simulink model "mmcs_s2f"  (R2021b)
settings: Solver=FixedStepDiscrete  StartTime=0.0  StopTime=5  FixedStep=T_HF_TASK  RelTol=1e-3  EnableMultiTasking=on
PostLoadFcn:
  | run('init.m')
values from neighbouring files (symbols this model uses):
  ALIGN_DURATION = 700.0    [mmcs_s2f_dd.sldd]
  ALIGN_FINAL_CURRENT = 3277.0    [mmcs_s2f_dd.sldd]
  ALIGN_FINAL_SPEED = 0.0    [mmcs_s2f_dd.sldd]
  ALIGN_INIT_CURRENT = 1638.0    [mmcs_s2f_dd.sldd]
  ALIGN_THETA = 2731.0    [mmcs_s2f_dd.sldd]
  AMPTOS16 = 3277.0    [mmcs_s2f_dd.sldd]
  DIVSQRT_3 = 18918.0    [mmcs_s2f_dd.sldd]
  ENC_PT_CTRL = 4.0    [mmcs_s2f_dd.sldd]
  ENC_PULSE_NUM = 4000    [mmcs_s2f_dd.sldd]
  ENC_ST_CTRL = 2.0    [mmcs_s2f_dd.sldd]
  IF_ACC_DURATION = 1500.0    [mmcs_s2f_dd.sldd]
  IF_FINAL_CURRENT = 3277.0    [mmcs_s2f_dd.sldd]
  IF_FINAL_CURRENT_LOL = -3277.0    [mmcs_s2f_dd.sldd]
  IF_FINAL_CURRENT_UPL = 3277.0    [mmcs_s2f_dd.sldd]
  IF_FINAL_SPEED = 600.0    [mmcs_s2f_dd.sldd]
  IF_FINAL_SPEED_LOL = -600.0    [mmcs_s2f_dd.sldd]
  IF_FINAL_SPEED_UPL = 600.0    [mmcs_s2f_dd.sldd]
  IF_INIT_CURRENT = 1638.0    [mmcs_s2f_dd.sldd]
  INT16_MAX = 32767.0    [mmcs_s2f_dd.sldd]
  INT16_MIN = -32768.0    [mmcs_s2f_dd.sldd]
  MOTOR_F = 7.0E-6    [mmcs_s2f_dd.sldd]
  MOTOR_J = 2.8E-6    [mmcs_s2f_dd.sldd]
  MOTOR_PN = 4    [mmcs_s2f_dd.sldd]
  MOTOR_PNF = 4.0    [mmcs_s2f_dd.sldd]
  MOTOR_TL = 0.001    [mmcs_s2f_dd.sldd]
  PI_KI_PLL : value not decoded    [mmcs_s2f_dd.sldd]
  PI_KI_POS : value not decoded    [mmcs_s2f_dd.sldd]
  PI_KI_SPD : value not decoded    [mmcs_s2f_dd.sldd]
  PI_KI_TQ : value not decoded    [mmcs_s2f_dd.sldd]
  PI_KP_PLL : value not decoded    [mmcs_s2f_dd.sldd]
  PI_KP_POS : value not decoded    [mmcs_s2f_dd.sldd]
  PI_KP_SPD : value not decoded    [mmcs_s2f_dd.sldd]
  PI_KP_TQ : value not decoded    [mmcs_s2f_dd.sldd]
  PWM_FREQUENCY = 10000.0    [mmcs_s2f_dd.sldd]
  PWM_PERIOD_CYCLES = 7200.0    [mmcs_s2f_dd.sldd]
  RAD2RPM_F_DEN = 1000.0    [mmcs_s2f_dd.sldd]
  RAD2RPM_F_NUM = 9549.0    [mmcs_s2f_dd.sldd]
  RADTOS16_F = 10430.378350470453    [mmcs_s2f_dd.sldd]
  RADTOS16_I = 10430.0    [mmcs_s2f_dd.sldd]
  REF_CURRENT_LOL = -11470.0    [mmcs_s2f_dd.sldd]
  REF_CURRENT_UPL = 11470.0    [mmcs_s2f_dd.sldd]
  STM_ALIGN = 4.0    [mmcs_s2f_dd.sldd]
  STM_IFRUN = 5.0    [mmcs_s2f_dd.sldd]
  STM_INIT = 1.0    [mmcs_s2f_dd.sldd]
  STM_PTRUN = 7.0    [mmcs_s2f_dd.sldd]
  STM_START = 12.0    [mmcs_s2f_dd.sldd]
  STM_STRUN = 6.0    [mmcs_s2f_dd.sldd]
  STM_SWITCH = 11.0    [mmcs_s2f_dd.sldd]
  STO_C1 = 588    [mmcs_s2f_dd.sldd]
  STO_C2 = -5703    [mmcs_s2f_dd.sldd]
  STO_C3 = 1554    [mmcs_s2f_dd.sldd]
  STO_C4 = 7484    [mmcs_s2f_dd.sldd]
  STO_C5 = 1831    [mmcs_s2f_dd.sldd]
  STO_EST_MAX = 134213632.0    [mmcs_s2f_dd.sldd]
  STO_EST_MIN = -134213632.0    [mmcs_s2f_dd.sldd]
  STO_F1 = 4096.0    [mmcs_s2f_dd.sldd]
  STO_F2 = 4096.0    [mmcs_s2f_dd.sldd]
  STO_ST_CTRL = 3.0    [mmcs_s2f_dd.sldd]
  STOMS = 1000.0    [mmcs_s2f_dd.sldd]
  T_HF_TASK = 0.0001    [mmcs_s2f_dd.sldd]
  T_MF_TASK = 0.002    [mmcs_s2f_dd.sldd]
  TORQ_CTRL = 0.0    [mmcs_s2f_dd.sldd]
  U32MAXdivPulseNumber = 1073741    [mmcs_s2f_dd.sldd]
  VBUS = 24.0    [mmcs_s2f_dd.sldd]
undefined symbols (not defined in the file or in its folder): DiscIntNeverNeededParam
libraries: simulink x22, slpidlib x5, mcbplantlib x1, autolibpmsmexterior x1
(part 4 of 5)

== system mmcs_s2f/MFTask/SpdCtrl/SpdControler ==
  reset : Inport  OutDataTypeStr=boolean
  spd_ref : Inport  Port=2
  spd_fed : Inport  Port=3
  Constant6 : Constant  Value=0  OutDataTypeStr=int16
  Data Type Conversion : DataTypeConversion  OutDataTypeStr=int16  RndMeth=Zero
  Scope : Scope  NumInputPorts=2
  SpdControler : slpidlib/PID Controller  Controller=PI  Form=Parallel  TimeDomain=Discrete-time  UseExternalTs=off  SampleTime=-1  IntegratorMethod=Forward Euler  FilterMethod=Forward Euler  ControllerParametersSource=internal  P=PI_KP_SPD  I=PI_KI_SPD  D=0  UseFilter=on  N=100  TunerSelectOption=Transfer Function Based (PID Tuner App)  InitialConditionSource=internal  InitialConditionForIntegrator=0  InitialConditionForFilter=0  DifferentiatorICPrevScaledInput=0  ExternalReset=level  TrackingMode=off  Kt=1  LimitOutput=on  SatLimitsSource=internal  UpperSaturationLimit=REF_CURRENT_UPL  LowerSaturationLimit=REF_CURRENT_LOL  LinearizeAsGain=off  AntiWindupMode=clamping  Kb=1  RndMeth=Zero  SaturateOnIntegerOverflow=on  PGainOutDataTypeStr=fixdt(1,32,11)  PProdOutDataTypeStr=fixdt(1,32,11)  POutMin=[]  POutMax=[]  IGainOutDataTypeStr=fixdt(1,32,11)  IProdOutDataTypeStr=fixdt(1,32,11)  IOutMin=[]  IOutMax=[]  DOutMin=[]  DOutMax=[]  NOutMin=[]  NOutMax=[]  SumOutDataTypeStr=int32  SumOutMin=[]  SumOutMax=[]  SaturationOutDataTypeStr=int32  SaturationOutMin=[]  SaturationOutMax=[]  PParamDataTypeStr=fixdt(1,32,16)  PParamMin=[]  PParamMax=[]  IParamDataTypeStr=fixdt(1,32,16)  IParamMin=[]  IParamMax=[]  DParamMin=[]  DParamMax=[]  NParamMin=[]  NParamMax=[]  KbParamMin=[]  KbParamMax=[]  KtParamMin=[]  KtParamMax=[]  KbOutMin=[]  KbOutMax=[]  KtOutMin=[]  KtOutMax=[]  IntegratorOutDataTypeStr=fixdt(1,32,11)  IntegratorOutMin=[]  IntegratorOutMax=[]  FilterOutMin=[]  FilterOutMax=[]  SumI1OutMin=[]  SumI1OutMax=[]  SumI2OutMin=[]  SumI2OutMax=[]  SumI3OutMin=[]  SumI3OutMax=[]  SumI4OutMin=[]  SumI4OutMax=[]  SumDOutMin=[]  SumDOutMax=[]  SumAccumDataTypeStr=fixdt(1,32,11)  DifferentiatorOutMin=[]  DifferentiatorOutMax=[]  FilterDiffOutCoefMin=[]  FilterDiffOutCoefMax=[]  ReciprocalOutMin=[]  ReciprocalOutMax=[]  SumDenOutMin=[]  SumDenOutMax=[]  SumNumOutMin=[]  SumNumOutMax=[]  DivideOutMin=[]  DivideOutMax=[]  UdiffTsProdOutMin=[]  UdiffTsProdOutMax=[]  NTsProdOutMin=[]  NTsProdOutMax=[]  UintegralTsProdOutMin=[]  UintegralTsProdOutMax=[]  UngainTsProdOutMin=[]  UngainTsProdOutMax=[]  IntegratorContinuousStateAttributes=''  IntegratorStateMustResolveToSignalObject=off  IntegratorRTWStateStorageClass=Auto  FilterContinuousStateAttributes=''  FilterStateMustResolveToSignalObject=off  FilterRTWStateStorageClass=Auto  ParallelPVariant=InternalParameters  IdealPVariant=Disabled  IVariant=InternalParameters  DVariant=Disabled  IntegratorVariant=Discrete  SatVariant=Enabled  AWVariant=DiscClampingParallel  PCopyVariant=Disabled  TRVariant=Disabled  FdbkBlocksVariant=Forward  IdealPFdbkVariant=Disabled  SatFdbkVariant=Disabled  DerivativeFilterVariant=Disabled  NVariant=Disabled  NCopyVariant=Disabled_SignalSpec  FilterICVariant=Disabled  IntegratorICVariant=InternalICs  ExternalResetVariant=ExternalReset  TRSumVariant=Passthrough  SumFdbkVariant=Disabled  SumVariant=Sum_PI  TsampFilterVariant=InternalTs  TsampNgainVariant=Passthrough  TsampIntegralVariant=Passthrough  ExternalSaturationOutDataTypeStr=Inherit: Same as second input
  Sum : Sum  Inputs=|+-  RndMeth=Zero
  id_ref : Outport  OutDataTypeStr=int16
  iq_ref : Outport  Port=2  OutDataTypeStr=int16
  spd_ramp : Outport  Port=3  OutDataTypeStr=int16
  wires:
  Constant6/1 -> id_ref/1
  Sum/1 -> SpdControler/1
  spd_ref/1 -> Scope/1, spd_ramp/1, Sum/1
  spd_fed/1 -> Sum/2, Scope/2
  SpdControler/1 -> Data Type Conversion/1
  Data Type Conversion/1 -> iq_ref/1
  reset/1 -> SpdControler/2

== system mmcs_s2f/MFTask/SysCtrlModeUpdDet/If Action Subsystem ==
  pos_fed : Inport  OutDataTypeStr=int32
  Action Port : ActionPort  ActionPortLabel=if(u1)
  Constant : Constant  Value=0  OutDataTypeStr=uint8
  Constant1 : Constant  Value=0  OutDataTypeStr=single
  Constant2 : Constant  Value=RADTOS16_F  OutDataTypeStr=single
  Data Store Write1 : DataStoreWrite  DataStoreName=pos_ctrl  DataStoreElements=pos_ctrl.final_angle#pos_ctrl.theta#pos_ctrl.tc_sts#pos_ctrl.elapse_time  IndexOptions=Index vector (dialog)  Indices=1  OutputSizes=1
  Divide : Product  Inputs=*/  OutDataTypeStr=single  RndMeth=Zero
  wires:
  pos_fed/1 -> Divide/1
  Constant/1 -> Data Store Write1/3
  Constant1/1 -> Data Store Write1/4
  Constant2/1 -> Divide/2
  Divide/1 -> Data Store Write1/2, Data Store Write1/1

== system mmcs_s2f/MFTask/TorqCtrl/AlignRamp ==
  reset : Inport  OutDataTypeStr=uint8
  Constant1 : Constant  Value=ALIGN_INIT_CURRENT  OutDataTypeStr=int16
  Constant5 : Constant  Value=ALIGN_FINAL_CURRENT  OutDataTypeStr=int16
  Constant6 : Constant  Value=0  OutDataTypeStr=int16
  Constant7 : Constant  Value=ALIGN_DURATION  OutDataTypeStr=uint16
  Constant9 : Constant  Value=ALIGN_FINAL_SPEED  OutDataTypeStr=int16
  IfControler : Subsystem
      settings: RTWFcnNameOpts=Use subsystem name  RTWFileNameOpts=Use subsystem name
  id_ref : Outport  OutDataTypeStr=int16
  iq_ref : Outport  Port=2  OutDataTypeStr=int16
  spd_ramp : Outport  Port=3  OutDataTypeStr=int16
  wires:
  IfControler/1(i_ref) -> id_ref/1
  Constant7/1 -> IfControler/4(duration_ms)
  Constant9/1 -> IfControler/3(final_spd)
  Constant6/1 -> iq_ref/1
  Constant5/1 -> IfControler/2(final_i)
  reset/1 -> IfControler/5(reset)
  Constant1/1 -> IfControler/1(init_i)
  IfControler/2(spd_ref) -> spd_ramp/1

== system mmcs_s2f/MFTask/TorqCtrl/AligntAction ==
  id_ref_i : Inport  OutDataTypeStr=int16
  iq_ref_i : Inport  Port=2  OutDataTypeStr=int16
  spd_ramp_i : Inport  Port=3  OutDataTypeStr=int16
  Action Port : ActionPort  ActionPortLabel=case [ 4 ]:
  id_ref : Outport  OutDataTypeStr=int16
  iq_ref : Outport  Port=2  OutDataTypeStr=int16
  spd_ramp : Outport  Port=3  OutDataTypeStr=int16
  wires:
  id_ref_i/1 -> id_ref/1
  spd_ramp_i/1 -> spd_ramp/1
  iq_ref_i/1 -> iq_ref/1

== system mmcs_s2f/MFTask/TorqCtrl/DefAction ==
  Action Port : ActionPort  ActionPortLabel=default:
  Constant : Constant  Value=0  OutDataTypeStr=int16
  Constant1 : Constant  Value=0  OutDataTypeStr=int16
  Constant2 : Constant  Value=0  OutDataTypeStr=int16
  id_ref : Outport  OutDataTypeStr=int16
  iq_ref : Outport  Port=2  OutDataTypeStr=int16
  spd_ramp : Outport  Port=3  OutDataTypeStr=int16
  wires:
  Constant2/1 -> spd_ramp/1
  Constant1/1 -> iq_ref/1
  Constant/1 -> id_ref/1

== system mmcs_s2f/MFTask/TorqCtrl/IFRamp ==
  reset : Inport  OutDataTypeStr=uint8
  spd_ref : Inport  Port=2  OutDataTypeStr=int16
  Constant1 : Constant  Value=IF_INIT_CURRENT  OutDataTypeStr=int16
  Constant5 : Constant  Value=IF_FINAL_CURRENT  OutDataTypeStr=int16
  Constant6 : Constant  Value=0  OutDataTypeStr=int16
  Constant7 : Constant  Value=IF_ACC_DURATION  OutDataTypeStr=uint16
  Constant9 : Constant  Value=IF_FINAL_SPEED  OutDataTypeStr=int16
  Demux : Demux  Outputs=3
      settings: DisplayOption=none
  Gain : Gain  Gain=-1  ParamDataTypeStr=int16  OutDataTypeStr=int16  RndMeth=Zero
  IfControler : Subsystem
      settings: RTWFcnNameOpts=Use subsystem name  RTWFileNameOpts=Use subsystem name
  Mux : Mux  Inputs=3
  Switch : Switch  RndMeth=Zero
  id_ref : Outport  OutDataTypeStr=int16
  iq_ref : Outport  Port=2  OutDataTypeStr=int16
  spd_ramp : Outport  Port=3  OutDataTypeStr=int16
  wires:
  spd_ref/1 -> Switch/2
  IfControler/2(spd_ref) -> spd_ramp/1
  Constant6/1 -> id_ref/1
  IfControler/1(i_ref) -> iq_ref/1
  Constant7/1 -> IfControler/4(duration_ms)
  reset/1 -> IfControler/5(reset)
  Gain/1 -> Switch/3
  Constant1/1 -> Mux/1
  Constant5/1 -> Mux/2
  Constant9/1 -> Mux/3
  Mux/1 -> Gain/1, Switch/1
  Switch/1 -> Demux/1
  Demux/2 -> IfControler/2(final_i)
  Demux/1 -> IfControler/1(init_i)
  Demux/3 -> IfControler/3(final_spd)

== system mmcs_s2f/MFTask/TorqCtrl/IFStart ==
  id_ref_i : Inport  OutDataTypeStr=int16
  iq_ref_i : Inport  Port=2  OutDataTypeStr=int16
  spd_ramp_i : Inport  Port=3  OutDataTypeStr=int16
  Action Port : ActionPort  ActionPortLabel=case [ 5 ]:
  id_ref : Outport  OutDataTypeStr=int16
  iq_ref : Outport  Port=2  OutDataTypeStr=int16
  spd_ramp : Outport  Port=3  OutDataTypeStr=int16
  wires:
  iq_ref_i/1 -> iq_ref/1
  spd_ramp_i/1 -> spd_ramp/1
  id_ref_i/1 -> id_ref/1

== system mmcs_s2f/HFTask/AngleCalc/VssCalcAngle/EncCalcAngle ==
  cnt : Inport  OutDataTypeStr=int32
  Constant : Constant  Value=65536  OutDataTypeStr=int32
  Constant6 : Constant  Value=U32MAXdivPulseNumber  OutDataTypeStr=uint32
  Data Type Conversion1 : DataTypeConversion  OutDataTypeStr=int16  RndMeth=Zero
  Data Type Conversion2 : DataTypeConversion  OutDataTypeStr=int16  RndMeth=Zero
  Divide : Product  Inputs=*/  OutDataTypeStr=int32  RndMeth=Zero
  Gain5 : Gain  Gain=MOTOR_PN  OutDataTypeStr=int32  RndMeth=Zero
  Product2 : Product  OutDataTypeStr=int64  RndMeth=Zero
  Scope : Scope  NumInputPorts=2
  theta_e : Outport  OutDataTypeStr=int16
  wires:
  Constant6/1 -> Product2/2
  Product2/1 -> Divide/1
  Data Type Conversion2/1 -> Scope/2, theta_e/1  "theta_e"
  cnt/1 -> Product2/1
  Constant/1 -> Divide/2
  Divide/1 -> Data Type Conversion1/1
  Gain5/1 -> Data Type Conversion2/1
  Data Type Conversion1/1 -> Scope/1, Gain5/1  "theta_m"

== system mmcs_s2f/HFTask/AngleCalc/VssCalcAngle/VssEncoder ==
  spd_ref : Inport  OutDataTypeStr=int16
  theta_0 : Inport  Port=2  OutDataTypeStr=int16
  reset : Inport  Port=3  OutDataTypeStr=uint8
  Add : Sum  RndMeth=Zero
  Constant1 : Constant  Value=60  OutDataTypeStr=uint8
  Constant7 : Constant  Value=ENC_PULSE_NUM  OutDataTypeStr=int32
  Discrete-Time Integrator1 : DiscreteIntegrator  ExternalReset=level  SampleTime=-1  OutDataTypeStr=int32  RndMeth=Zero  ICPrevOutput=DiscIntNeverNeededParam  ICPrevScaledInput=DiscIntNeverNeededParam
  Divide : Product  Inputs=*/  OutDataTypeStr=int32  RndMeth=Zero
  Math Function : Math  Operator=rem  SaturateOnIntegerOverflow=on
  Product1 : Product  OutDataTypeStr=int32  RndMeth=Zero
  enc_cnt : Outport
  wires:
  spd_ref/1 -> Product1/1
  Constant7/1 -> Product1/2, Math Function/2
  Product1/1 -> Discrete-Time Integrator1/1
  Math Function/1 -> enc_cnt/1
  Discrete-Time Integrator1/1 -> Divide/1
  Divide/1 -> Add/1
  Add/1 -> Math Function/1
  theta_0/1 -> Add/2
  Constant1/1 -> Divide/2
  reset/1 -> Discrete-Time Integrator1/2

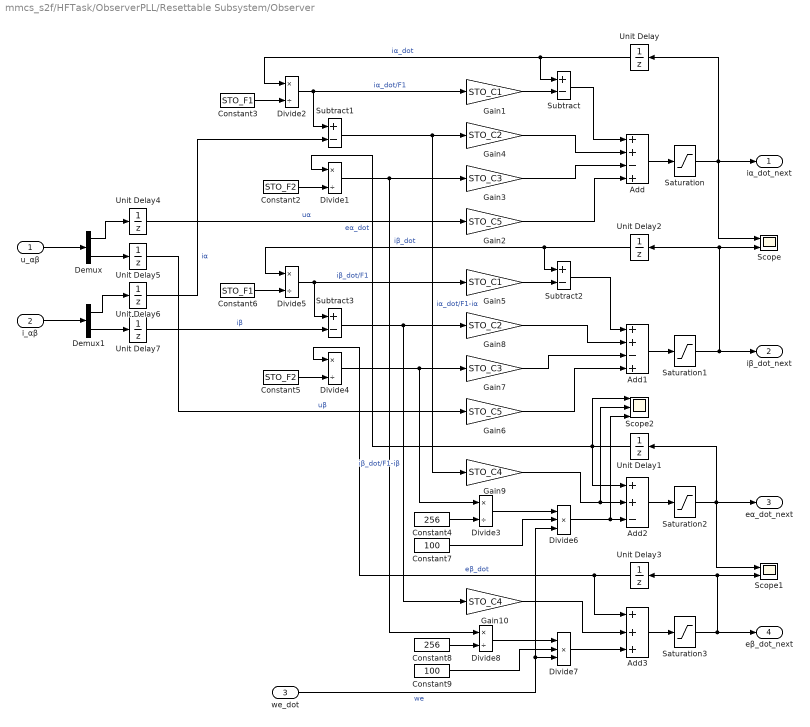
== system mmcs_s2f/HFTask/ObserverPLL/Resettable Subsystem/Observer ==
  u_αβ : Inport  OutDataTypeStr=int16
  i_αβ : Inport  Port=2  OutDataTypeStr=int16
  we_dot : Inport  Port=3  OutDataTypeStr=int16
  Add : Sum  Inputs=++-+  OutDataTypeStr=int32  RndMeth=Zero
  Add1 : Sum  Inputs=++-+  OutDataTypeStr=int32  RndMeth=Zero
  Add2 : Sum  Inputs=++-  OutDataTypeStr=int32  RndMeth=Zero
  Add3 : Sum  Inputs=+++  OutDataTypeStr=int32  RndMeth=Zero
  Constant2 : Constant  Value=STO_F2  OutDataTypeStr=int16
  Constant3 : Constant  Value=STO_F1  OutDataTypeStr=int16
  Constant4 : Constant  Value=256  OutDataTypeStr=int16
  Constant5 : Constant  Value=STO_F2  OutDataTypeStr=int16
  Constant6 : Constant  Value=STO_F1  OutDataTypeStr=int16
  Constant7 : Constant  Value=100  OutDataTypeStr=int16
  Constant8 : Constant  Value=256  OutDataTypeStr=int16
  Constant9 : Constant  Value=100  OutDataTypeStr=int16
  Demux : Demux  Outputs=2
      settings: DisplayOption=none
  Demux1 : Demux  Outputs=2
      settings: DisplayOption=none
  Divide{1..5,8} (6 alike) : Product  Inputs=*/  OutDataTypeStr=int32  RndMeth=Zero
  Divide6 : Product  Inputs=***  OutDataTypeStr=int32  RndMeth=Zero
  Divide7 : Product  Inputs=***  OutDataTypeStr=int32  RndMeth=Zero
  Gain1 : Gain  Gain=STO_C1  ParamDataTypeStr=int32  OutDataTypeStr=int32  RndMeth=Zero
  Gain10 : Gain  Gain=STO_C4  ParamDataTypeStr=int32  OutDataTypeStr=int32  RndMeth=Zero
  Gain2 : Gain  Gain=STO_C5  ParamDataTypeStr=int32  OutDataTypeStr=int32  RndMeth=Zero
  Gain3 : Gain  Gain=STO_C3  ParamDataTypeStr=int32  OutDataTypeStr=int32  RndMeth=Zero
  Gain4 : Gain  Gain=STO_C2  ParamDataTypeStr=int32  OutDataTypeStr=int32  RndMeth=Zero
  Gain5 : Gain  Gain=STO_C1  ParamDataTypeStr=int32  OutDataTypeStr=int32  RndMeth=Zero
  Gain6 : Gain  Gain=STO_C5  ParamDataTypeStr=int32  OutDataTypeStr=int32  RndMeth=Zero
  Gain7 : Gain  Gain=STO_C3  ParamDataTypeStr=int32  OutDataTypeStr=int32  RndMeth=Zero
  Gain8 : Gain  Gain=STO_C2  ParamDataTypeStr=int32  OutDataTypeStr=int32  RndMeth=Zero
  Gain9 : Gain  Gain=STO_C4  ParamDataTypeStr=int32  OutDataTypeStr=int32  RndMeth=Zero
  Saturation{,1..3} (4 alike) : Saturate  UpperLimit=STO_EST_MAX  LowerLimit=STO_EST_MIN  RndMeth=Zero
  Scope : Scope  NumInputPorts=2
  Scope1 : Scope  NumInputPorts=2
  Scope2 : Scope  NumInputPorts=3
  Subtract{,1..3} (4 alike) : Sum  Inputs=+-  OutDataTypeStr=int32  RndMeth=Zero
  Unit Delay{,1..7} (8 alike) : UnitDelay  SampleTime=-1  HasFrameUpgradeWarning=on
  iα_dot_next : Outport  OutDataTypeStr=int32
  iβ_dot_next : Outport  Port=2  OutDataTypeStr=int32
  eα_dot_next : Outport  Port=3  OutDataTypeStr=int32
  eβ_dot_next : Outport  Port=4  OutDataTypeStr=int32
  wires:
  Add/1 -> Saturation/1
  Unit Delay/1 -> Divide2/1, Subtract/1  "iα_dot"
  Add3/1 -> Saturation3/1
  Add2/1 -> Saturation2/1
  Demux/1 -> Unit Delay4/1
  Demux1/1 -> Unit Delay6/1
  Demux/2 -> Unit Delay5/1
  Demux1/2 -> Unit Delay7/1
  we_dot/1 -> Divide7/3, Divide6/3  "we"
  Unit Delay4/1 -> Gain2/1  "uα"
  Unit Delay6/1 -> Subtract1/2  "iα"
  u_αβ/1 -> Demux/1
  i_αβ/1 -> Demux1/1
  Gain2/1 -> Add/4
  Gain1/1 -> Subtract/2
  Subtract/1 -> Add/1
  Unit Delay1/1 -> Scope2/1, Divide1/1, Add2/1  "eα_dot"
  Constant2/1 -> Divide1/2
  Divide1/1 -> Gain3/1, Divide8/1
  Constant3/1 -> Divide2/2
  Divide2/1 -> Subtract1/1, Gain1/1  "iα_dot/F1"
  Subtract1/1 -> Gain4/1, Gain9/1  "iα_dot/F1-iα"
  Gain4/1 -> Add/2
  Gain6/1 -> Add1/4
  Unit Delay2/1 -> Divide5/1, Subtract2/1  "iβ_dot"
  Divide5/1 -> Subtract3/1, Gain5/1  "iβ_dot/F1"
  Constant6/1 -> Divide5/2
  Subtract3/1 -> Gain8/1, Gain10/1  "iβ_dot/F1-iβ"
  Gain8/1 -> Add1/2
  Constant5/1 -> Divide4/2
  Gain5/1 -> Subtract2/2
  Subtract2/1 -> Add1/1
  Add1/1 -> Saturation1/1
  Unit Delay5/1 -> Gain6/1  "uβ"
  Unit Delay7/1 -> Subtract3/2  "iβ"
  Unit Delay3/1 -> Divide4/1, Add3/1  "eβ_dot"
  Divide4/1 -> Gain7/1, Divide3/1
  Gain9/1 -> Add2/2, Scope2/2
  Gain10/1 -> Add3/2
  Divide6/1 -> Scope2/3, Add2/3
  Divide7/1 -> Add3/3
  Saturation/1 -> iα_dot_next/1, Scope/1, Unit Delay/1
  Saturation1/1 -> iβ_dot_next/1, Unit Delay2/1, Scope/2
  Saturation2/1 -> Scope1/1, eα_dot_next/1, Unit Delay1/1
  Saturation3/1 -> Unit Delay3/1, Scope1/2, eβ_dot_next/1
  Gain7/1 -> Add1/3
  Constant4/1 -> Divide3/2
  Divide3/1 -> Divide6/1
  Constant7/1 -> Divide6/2
  Gain3/1 -> Add/3
  Constant8/1 -> Divide8/2
  Divide8/1 -> Divide7/1
  Constant9/1 -> Divide7/2
